simulink model "sm_pulleys_xytable_cross"  (R2026a)
settings: Solver=VariableStepAuto  StopTime=13  EnableMultiTasking=on
model workspace (MATLAB code in the model file):
  | % Pulley parameters
  | p_th  = 0.01;
  | p_gd  = 0.005;
  | p_ga  = 25;
  | p_hr  = 0.005;
  | p_rho = 7000;
  | 
  | rad_drive = 0.015*2;
  | rad_axis = 0.015*2;
  | rad_ctr = 0.015;
  | 
  | % Platform parameters
  | t_base_l = 0.4;
  | t_base_w = 0.1;
  | t_base_h = 0.01;
  | 
  | t_slider_l = 0.15;
  | t_slider_w = 0.1;
  | t_slider_h = 0.01;
  | 
  | t_pos_l = 0.025;
  | t_pos_w = 0.45;
  | t_pos_h = 0.01;
  | 
  | t_base_clr = [0.5412 0.6824 0.8392];
  | t_slider_clr = [0.635 0.984 0.498];
  | t_pos_clr = [1.0 0.99607843 0.8];
  | 
  | p_drive_clr = t_base_clr*0.8;
  | p_axis_clr = t_pos_clr*0.8;
  | p_ctr_clr = t_slider_clr*0.8;
  | 
  | 
  | 
  | p_pos_off = 0.01;
undefined symbols (not defined in the file or in its folder): Local, X, Y, Z
libraries: sm_lib x48, Multibody_Parts_Lib x15, nesl_utility x13
(part 1 of 2)
CloseFcn:
  | try,close(h1_sm_pulleys_xytable_cross),end
  | clear h1_sm_pulleys_xytable_cross
  | try,close(h2_sm_pulleys_xytable_cross),end
  | clear h2_sm_pulleys_xytable_cross
  | try,close(h3_sm_pulleys_xytable_cross),end
  | clear h3_sm_pulleys_xytable_cross
  | try,close(h4_sm_pulleys_xytable_cross),end
  | clear h4_sm_pulleys_xytable_cross
  | 
  | 
  | clear simlog_sm_pulleys_xytable_cross
  | clear logsout_sm_pulleys_xytable_cross
Description:
  | Cable-Driven XY Table with Cross Base
  | 
  | Copyright 2026 The MathWorks, Inc.
settings Model: Creator=smiller  LastModifiedBy=smiller
settings DataIOCC: SignalLoggingName=logsout_sm_pulleys_xytable_cross
settings DebuggingCC: PregeneratedLibrarySubsystemCodeDiagnostic=none
settings SimscapeCC: SimscapeNominalValues="[{\"value\":\"10\",\"unit\":\"V\"},{\"value\":\"1\",\"unit\":\"A\"},{\"value\":\"10\",\"unit\":\"N*m\"},{\"value\":\"10\",\"unit\":\"bar\"},{\"value\":\"100\",\"unit\":\"kJ/kg\"},{\"value\":\"1\",\"unit\":\"kW\"},{\"value\":\"300\",\"unit\":\"K\"},{\"value\":\"100\",\"unit\":\"cm^3/s\"},{\"value\":\"1\",\"unit\":\"kN\"},{\"value\":\"1\",\"unit\":\"g/cm^3\"},{\"value\":\"1\",\"unit\":\"l\"},{\"value\":\"1\",\"unit\":\"cm^2\"},{\"value\":\"60\",\"unit\":\"Hz\"}]"  SimscapeLogSimulationStatistics=on  SimscapeLogName=simlog_sm_pulleys_xytable_cross
settings ConfigurationSet: Description=SimMechanics 2G
settings ExplorerConfigSet: InternalSimMechanicsExplorerSettings="<ExplorerConfiguration><canonicalview>aerospace</canonicalview><AnimationSetting><BasePlaybackSpeed>1.0</BasePlaybackSpeed><PlaybackSpeedFactor>1.0</PlaybackSpeedFactor></AnimationSetting><TilePanel><TileInfo><Tiles Columns=\"1\" Count=\"2\" Rows=\"2\"><Column Weight=\"1\"/><Row Weight=\"0.6424\"/><Row Weight=\"0.3576\"/><Tile Height=\"1\" Width=\"1\" X=\"0\" Y=\"0\"/><Tile Height=\"1\" Width=\"1\" X=\"0\" Y=\"1\"/></Tiles></TileInfo><SceneInfo><SceneViewer><BGColor><R>1</R><G>1</G><B>1</B></BGColor><Camera><DoPerspective>off</DoPerspective><Position><X>1.85532256000346015e-05</X><Y>-0.00427343685538296436</Y><Z>1.02990794223546889</Z></Position><Center><X>7.04853169139587633e-06</X><Y>0.00254160839863069388</Y><Z>0.0299311649922031596</Z></Center><Up><X>0.00283398063646299022</X><Y>0.999972761893709983</Y><Z>0.00681498528375228379</Z></Up><ViewLimDist>1</ViewLimDist><YLim>0.234492363482713712</YLim><XLim>0.277049961210973916</XLim></Camera></SceneViewer><SceneViewer><BGColor><R>1</R><G>1</G><B>1</B></BGColor><Camera><DoPerspective>off</DoPerspective><Position><X>-0.689691226810977609</X><Y>-0.584891014214740101</Y><Z>0.428792646519957021</Z></Position><Center><X>0.00287853310714154473</X><Y>0.0117733409261104611</Y><Z>0.0234054551197957761</Z></Center><Up><X>0.265483592004607194</X><Y>0.311705662060663302</Y><Z>0.912336584060759237</Z></Up><ViewLimDist>1</ViewLimDist><YLim>0.103903868048192807</YLim><XLim>0.221775141309421386</XLim></Camera></SceneViewer></SceneInfo></TilePanel><MechEditorPanel><Cameras/><GfxPanelCameraMap/><VideoCreator><PlaybackSpeedRatio>1.0</PlaybackSpeedRatio><FrameRate>30</FrameRate><VideoFormat>Motion JPEG AVI</VideoFormat><FrameSize>auto</FrameSize></VideoCreator></MechEditorPanel></ExplorerConfiguration>"

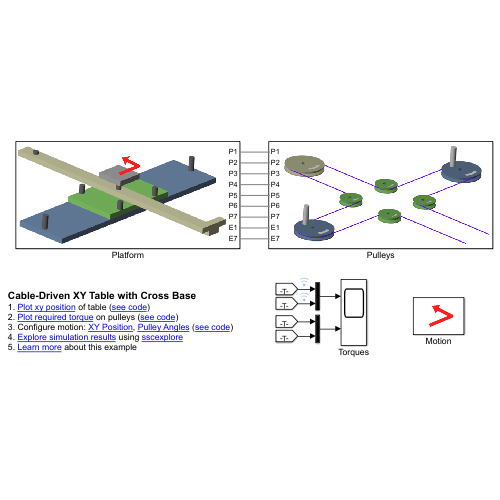
[thumbnail: Simulink's stored preview of the top-level diagram]
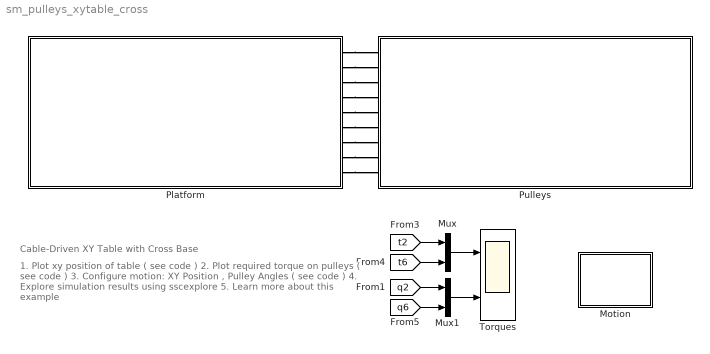
== system sm_pulleys_xytable_cross ==
  note: Cable-Driven XY Table with Cross Base
  note: 1. Plot xy position of table ( see code )
      | 2. Plot required torque on pulleys ( see code )
      | 3. Configure motion: XY Position , Pulley Angles ( see code )
      | 4. Explore simulation results using sscexplore
      | 5. Learn more about this example
  Motion : Subsystem
      mask Display: image('sm_pulleys_xytable_cross_motionXYMotion_IMAGE.png');
  Mux : Mux  Inputs=2
  Mux1 : Mux  Inputs=2
  Platform : Subsystem  Tag=PublishSubsystem
      mask Display: image('sm_pulleys_xytable_cross_platformXYMotion_IMAGE.png');
  Pulleys : Subsystem  Tag=PublishSubsystem
      mask Display: image('sm_pulleys_xytable_cross_pulleys_IMAGE.png');
  Torques : Scope  NumInputPorts=2
      settings: ActiveDisplayYMinimum=-0.14527  ActiveDisplayYMaximum=0.11195
  wires:
  [t2] -> Mux/1
  [t6] -> Mux/2
  [q2] -> Mux1/1
  [q6] -> Mux1/2
  Mux/1 -> Torques/1
  Mux1/1 -> Torques/2
  connections:
  Platform/RConn1 -- Pulleys/LConn1
  Platform/RConn2 -- Pulleys/LConn2
  Platform/RConn3 -- Pulleys/LConn3
  Platform/RConn4 -- Pulleys/LConn4
  Platform/RConn5 -- Pulleys/LConn5
  Platform/RConn6 -- Pulleys/LConn6
  Platform/RConn7 -- Pulleys/LConn7
  Platform/RConn8 -- Pulleys/LConn8
  Platform/RConn9 -- Pulleys/LConn9

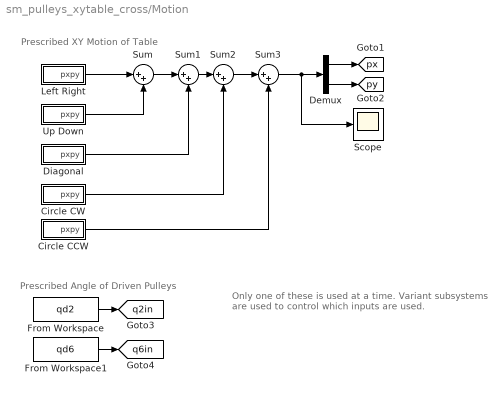
== system sm_pulleys_xytable_cross/Motion ==
  note: Only one of these is used at a time. Variant subsystems are used to control which inputs are used.
  note: Prescribed Angle of Driven Pulleys
  note: Prescribed XY Motion of Table
  Circle CCW : Subsystem
  Circle CW : Subsystem
  Demux : Demux  Outputs=2
  Diagonal : Subsystem
  From Workspace : FromWorkspace  VariableName=qd2
  From Workspace1 : FromWorkspace  VariableName=qd6
  Left Right : Subsystem
  Scope : Scope
      settings: ActiveDisplayYMinimum=-0.125  ActiveDisplayYMaximum=0.125
  Sum{,1..3} (4 alike) : Sum  Inputs=|++
  Up Down : Subsystem
  tag scope: px=global, py=global, q2in=global, q6in=global
  wires:
  Demux/1 -> [px]
  Demux/2 -> [py]
  Sum3/1 -> Scope/1, Demux/1
  Left Right/1(pxpy) -> Sum/1
  Diagonal/1(pxpy) -> Sum1/2
  Sum/1 -> Sum1/1
  Up Down/1(pxpy) -> Sum/2
  Sum1/1 -> Sum2/1
  Circle CW/1(pxpy) -> Sum2/2
  From Workspace/1 -> [q2in]
  From Workspace1/1 -> [q6in]
  Sum2/1 -> Sum3/1
  Circle CCW/1(pxpy) -> Sum3/2

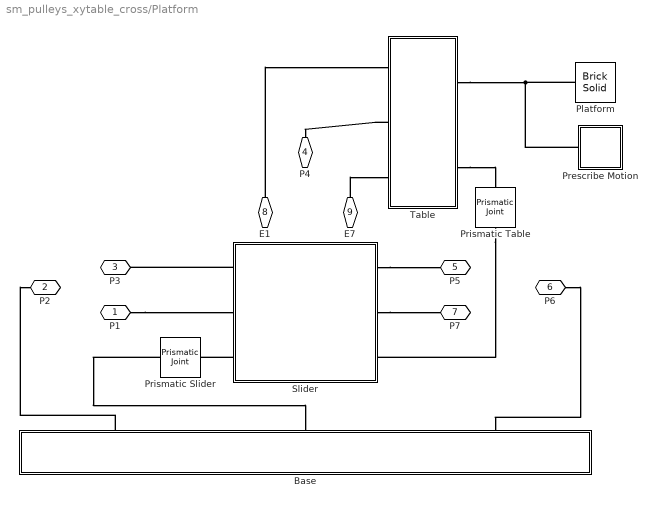
== system sm_pulleys_xytable_cross/Platform ==
  Base : Subsystem
      mask Display: image('sm_pulleys_xytable_cross_base_IMAGE.png');
  Platform : sm_lib/Body Elements/Brick Solid  BrickDimensions=[0.05 0.05 0.01]  BrickDimensionsUnits=m  ExportEntireGeometry=off  InertiaType=CalculateFromGeometry  BasedOnType=Density  Density=1000  DensityUnits=kg/m^3  Mass=1  MassUnits=kg  CenterOfMass=[0 0 0]  CenterOfMassUnits=m  MomentsOfInertia=[1 1 1]  MomentsOfInertiaUnits=kg*m^2  ProductsOfInertia=[0 0 0]  ProductsOfInertiaUnits=kg*m^2  GraphicType=FromGeometry  MarkerShape=Sphere  MarkerSize=10  GraphicVisPropType=SimpleVisualProperties  GraphicDiffuseColor=[0.8 0.8 0.8]  GraphicOpacity=1.0  GraphicSpecularColor=[0.5 0.5 0.5 1.0]  GraphicAmbientColor=[0.15 0.15 0.15 1.0]  GraphicEmissiveColor=[0.0 0.0 0.0 1.0]  GraphicShininess=75  DoExposeReferenceFrame=off  SerializedFrames=<Frames><Frame><Id>Frame1</Id><Value><Name>T</Name><Origin><Source>GeometricFeature</Source><FeatureName>+z surface</FeatureName></Origin><PrimaryAxis><DefinedDirection>+Z</DefinedDirection><Source>ReferenceFrame</Source><SourceDirection>+Z</SourceDirection><FeatureName></FeatureName></PrimaryAxis><SecondaryAxis><DefinedDirection>+X</DefinedDirection><Source>ReferenceFrame</Source><SourceDirection>+X</SourceDirection><FeatureName></FeatureName></SecondaryAxis></Value></Frame><Frame><Id>Frame2</Id><Value><Name>B</Name><Origin><Source>GeometricFeature</Source><FeatureName>-z surface</FeatureName></Origin><PrimaryAxis><DefinedDirection>+Z</DefinedDirection><Source>ReferenceFrame</Source><SourceDirection>+Z</SourceDirection><FeatureName></FeatureName></PrimaryAxis><SecondaryAxis><DefinedDirection>+X</DefinedDirection><Source>ReferenceFrame</Source><SourceDirection>+X</SourceDirection><FeatureName></FeatureName></SecondaryAxis></Value></Frame></Frames>
  Prescribe Motion : Subsystem  Variant=on  VariantControlMode=label  VariantControl=Variant1  LabelModeActiveChoice=On
      settings: AttributesFormatString=%<ActiveVariant>
      mask Display:
      | blk = Multibody_Parts_Library_activeVariantBlock(gcb);
      | eval(get_param(blk, 'MaskDisplay'));
  Prismatic Table : sm_lib/Joints/Prismatic Joint  JointMode=Normal  CompositeWrenchDir=FollowerOnBase  CompositeWrenchFrame=BaseFrame  SenseConstraintForce=off  SenseConstraintTorque=off  SenseTotalForce=off  SenseTotalTorque=off  PositionTargetSpecify=off  PositionTargetPriority=High  PositionTargetValue=0  PositionTargetValueUnits=m  VelocityTargetSpecify=off  VelocityTargetPriority=High  VelocityTargetValue=0  VelocityTargetValueUnits=m/s  EquilibriumPosition=0  EquilibriumPositionUnits=m  SpringStiffness=0  SpringStiffnessUnits=N/m  DampingCoefficient=0  DampingCoefficientUnits=N/(m/s)  LowerLimitSpecify=off  LowerLimitBound=-1  LowerLimitBoundUnits=m  LowerLimitStiffness=1e6  LowerLimitStiffnessUnits=N/m  LowerLimitDamping=1e3  LowerLimitDampingUnits=N/(m/s)  LowerLimitTransitionRegionWidth=1e-4  LowerLimitTransitionRegionWidthUnits=m  UpperLimitSpecify=off  UpperLimitBound=1  UpperLimitBoundUnits=m  UpperLimitStiffness=1e6  UpperLimitStiffnessUnits=N/m  UpperLimitDamping=1e3  UpperLimitDampingUnits=N/(m/s)  UpperLimitTransitionRegionWidth=1e-4  UpperLimitTransitionRegionWidthUnits=m  TorqueActuationMode=NoTorque  MotionActuationMode=ComputedMotion  SensePosition=off  SenseVelocity=off  SenseAcceleration=off  SenseTorqueForce=off  SenseLowerLimitTorqueForce=off  SenseUpperLimitTorqueForce=off
  Prismatic Slider : sm_lib/Joints/Prismatic Joint  JointMode=Normal  CompositeWrenchDir=FollowerOnBase  CompositeWrenchFrame=BaseFrame  SenseConstraintForce=off  SenseConstraintTorque=off  SenseTotalForce=off  SenseTotalTorque=off  PositionTargetSpecify=off  PositionTargetPriority=High  PositionTargetValue=0  PositionTargetValueUnits=m  VelocityTargetSpecify=off  VelocityTargetPriority=High  VelocityTargetValue=0  VelocityTargetValueUnits=m/s  EquilibriumPosition=0  EquilibriumPositionUnits=m  SpringStiffness=0  SpringStiffnessUnits=N/m  DampingCoefficient=0  DampingCoefficientUnits=N/(m/s)  LowerLimitSpecify=off  LowerLimitBound=-1  LowerLimitBoundUnits=m  LowerLimitStiffness=1e6  LowerLimitStiffnessUnits=N/m  LowerLimitDamping=1e3  LowerLimitDampingUnits=N/(m/s)  LowerLimitTransitionRegionWidth=1e-4  LowerLimitTransitionRegionWidthUnits=m  UpperLimitSpecify=off  UpperLimitBound=1  UpperLimitBoundUnits=m  UpperLimitStiffness=1e6  UpperLimitStiffnessUnits=N/m  UpperLimitDamping=1e3  UpperLimitDampingUnits=N/(m/s)  UpperLimitTransitionRegionWidth=1e-4  UpperLimitTransitionRegionWidthUnits=m  TorqueActuationMode=NoTorque  MotionActuationMode=ComputedMotion  SensePosition=off  SenseVelocity=off  SenseAcceleration=off  SenseTorqueForce=off  SenseLowerLimitTorqueForce=off  SenseUpperLimitTorqueForce=off
  Slider : Subsystem
      mask Display: image('sm_pulleys_xytable_cross_slider_IMAGE.png');
  Table : Subsystem
      mask Display: image('sm_pulleys_xytable_cross_table_IMAGE.png')
  P1 : PMIOPort  Side=Right
  P2 : PMIOPort  Port=2  Side=Right
  P3 : PMIOPort  Port=3  Side=Right
  P4 : PMIOPort  Port=4  Side=Right
  P5 : PMIOPort  Port=5  Side=Right
  P6 : PMIOPort  Port=6  Side=Right
  P7 : PMIOPort  Port=7  Side=Right
  E1 : PMIOPort  Port=8  Side=Right
  E7 : PMIOPort  Port=9  Side=Right
  connections:
  E1/RConn1 -- Table/LConn1
  E7/RConn1 -- Table/LConn3
  Table/LConn2 -- P4/RConn1
  Table/RConn2 -- Prismatic Table/RConn1
  Prismatic Table/LConn1 -- Slider/RConn3
  Slider/LConn3 -- Prismatic Slider/RConn1
  P1/RConn1 -- Slider/LConn2
  Prismatic Slider/LConn1 -- Base/RConn2
  P6/RConn1 -- Base/RConn3
  Slider/RConn1 -- P5/RConn1
  Slider/LConn1 -- P3/RConn1
  Slider/RConn2 -- P7/RConn1
  Base/RConn1 -- P2/RConn1
  Platform/RConn1 -- Table/RConn1 -- Prescribe Motion/RConn1

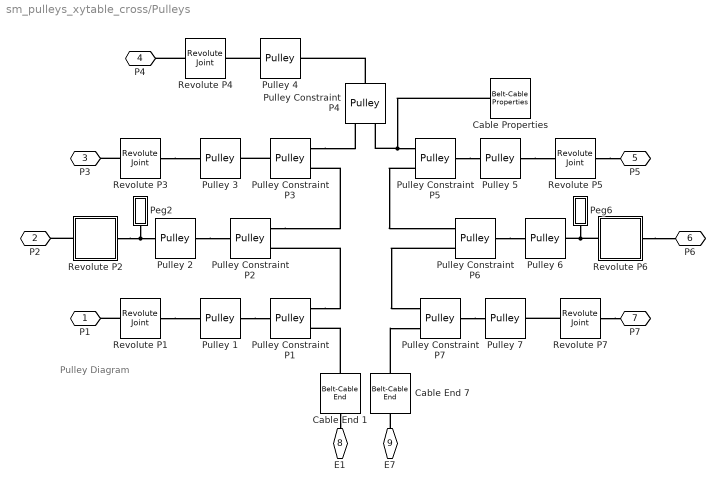
== system sm_pulleys_xytable_cross/Pulleys ==
  note: Pulley
      | Diagram
  Cable End 1 : sm_lib/Belts and Cables/Belt-Cable End
  Cable End 7 : sm_lib/Belts and Cables/Belt-Cable End
  Cable Properties : sm_lib/Belts and Cables/Belt-Cable Properties  DrumBeltCableAlignment=MonitoredPlanar  GraphicType=PitchLine  GraphicVisPropType=SimpleVisualProperties  GraphicDiffuseColor=[0.4 0.0 1.0]  GraphicOpacity=1.0  GraphicSpecularColor=[0.5 0.5 0.5 1.0]  GraphicAmbientColor=[0.15 0.15 0.15 1.0]  GraphicEmissiveColor=[0.0 0.0 0.0 1.0]  GraphicShininess=75
  Peg2 : Subsystem
  Peg6 : Subsystem
  Pulley Constraint P{1,3,5,7} (4 alike) : sm_lib/Belts and Cables/Pulley  PitchRadius=rad_ctr  PitchRadiusUnits=m  InitialWrapAngleLowerBound=0.0  InitialWrapAngleLowerBoundUnits=deg  SenseWrapAngle=off  SensePulleyAngleA=off  SensePulleyAngleB=off  SenseFleetAngleA=off  SenseFleetAngleB=off
  Pulley Constraint P2 : sm_lib/Belts and Cables/Pulley  PitchRadius=rad_drive  PitchRadiusUnits=m  InitialWrapAngleLowerBound=0.0  InitialWrapAngleLowerBoundUnits=deg  SenseWrapAngle=off  SensePulleyAngleA=off  SensePulleyAngleB=off  SenseFleetAngleA=off  SenseFleetAngleB=off
  Pulley Constraint P4 : sm_lib/Belts and Cables/Pulley  PitchRadius=rad_axis  PitchRadiusUnits=m  InitialWrapAngleLowerBound=0.0  InitialWrapAngleLowerBoundUnits=deg  SenseWrapAngle=off  SensePulleyAngleA=off  SensePulleyAngleB=off  SenseFleetAngleA=off  SenseFleetAngleB=off
  Pulley Constraint P6 : sm_lib/Belts and Cables/Pulley  PitchRadius=rad_drive  PitchRadiusUnits=m  InitialWrapAngleLowerBound=0.0  InitialWrapAngleLowerBoundUnits=deg  SenseWrapAngle=off  SensePulleyAngleA=off  SensePulleyAngleB=off  SenseFleetAngleA=off  SenseFleetAngleB=off
  Pulley 1 : Multibody_Parts_Lib/Basic/Pulley  pulley_rad=rad_ctr  pulley_d_grv=p_gd  pulley_a_grv=p_ga  pulley_th=p_th  pulley_radh=p_hr  pulley_rho=p_rho  pulley_clr=p_ctr_clr  pulley_opc=1  pulley_zori=Yes, about X  popup_markings=One  mark_radius_range=[0.7 0.9]  mark_angle_range=60  mark_color=[1 1 1]
      settings: SourceProductName=Simscape Multibody Parts Library
  Pulley 2 : Multibody_Parts_Lib/Basic/Pulley  pulley_rad=rad_drive  pulley_d_grv=p_gd  pulley_a_grv=p_ga  pulley_th=p_th  pulley_radh=p_hr  pulley_rho=p_rho  pulley_clr=p_drive_clr  pulley_opc=1  pulley_zori=No  popup_markings=One  mark_radius_range=[0.7 0.9]  mark_angle_range=60  mark_color=[1 1 1]
      settings: SourceProductName=Simscape Multibody Parts Library
  Pulley 3 : Multibody_Parts_Lib/Basic/Pulley  pulley_rad=rad_ctr  pulley_d_grv=p_gd  pulley_a_grv=p_ga  pulley_th=p_th  pulley_radh=p_hr  pulley_rho=p_rho  pulley_clr=p_ctr_clr  pulley_opc=1  pulley_zori=Yes, about X  popup_markings=One  mark_radius_range=[0.7 0.9]  mark_angle_range=60  mark_color=[1 1 1]
      settings: SourceProductName=Simscape Multibody Parts Library
  Pulley 4 : Multibody_Parts_Lib/Basic/Pulley  pulley_rad=rad_axis  pulley_d_grv=p_gd  pulley_a_grv=p_ga  pulley_th=p_th  pulley_radh=p_hr  pulley_rho=p_rho  pulley_clr=p_axis_clr  pulley_opc=1  pulley_zori=Yes, about X  popup_markings=One  mark_radius_range=[0.7 0.9]  mark_angle_range=60  mark_color=[1 1 1]
      settings: SourceProductName=Simscape Multibody Parts Library
  Pulley 5 : Multibody_Parts_Lib/Basic/Pulley  pulley_rad=rad_ctr  pulley_d_grv=p_gd  pulley_a_grv=p_ga  pulley_th=p_th  pulley_radh=p_hr  pulley_rho=p_rho  pulley_clr=p_ctr_clr  pulley_opc=1  pulley_zori=No  popup_markings=One  mark_radius_range=[0.7 0.9]  mark_angle_range=60  mark_color=[1 1 1]
      settings: SourceProductName=Simscape Multibody Parts Library
  Pulley 6 : Multibody_Parts_Lib/Basic/Pulley  pulley_rad=rad_drive  pulley_d_grv=p_gd  pulley_a_grv=p_ga  pulley_th=p_th  pulley_radh=p_hr  pulley_rho=p_rho  pulley_clr=p_drive_clr  pulley_opc=1  pulley_zori=Yes, about X  popup_markings=One  mark_radius_range=[0.7 0.9]  mark_angle_range=60  mark_color=[1 1 1]
      settings: SourceProductName=Simscape Multibody Parts Library
  Pulley 7 : Multibody_Parts_Lib/Basic/Pulley  pulley_rad=rad_ctr  pulley_d_grv=p_gd  pulley_a_grv=p_ga  pulley_th=p_th  pulley_radh=p_hr  pulley_rho=p_rho  pulley_clr=p_ctr_clr  pulley_opc=1  pulley_zori=No  popup_markings=One  mark_radius_range=[0.7 0.9]  mark_angle_range=60  mark_color=[1 1 1]
      settings: SourceProductName=Simscape Multibody Parts Library
  Revolute P{1,3..5,7} (5 alike) : sm_lib/Joints/Revolute Joint  JointMode=Normal  CompositeWrenchDir=FollowerOnBase  CompositeWrenchFrame=BaseFrame  SenseConstraintForce=off  SenseConstraintTorque=off  SenseTotalForce=off  SenseTotalTorque=off  PositionTargetSpecify=off  PositionTargetPriority=High  PositionTargetValue=0  PositionTargetValueUnits=deg  VelocityTargetSpecify=off  VelocityTargetPriority=High  VelocityTargetValue=0  VelocityTargetValueUnits=deg/s  EquilibriumPosition=0  EquilibriumPositionUnits=deg  SpringStiffness=0  SpringStiffnessUnits=N*m/deg  DampingCoefficient=0  DampingCoefficientUnits=N*m/(deg/s)  LowerLimitSpecify=off  LowerLimitBound=-90  LowerLimitBoundUnits=deg  LowerLimitStiffness=1e4  LowerLimitStiffnessUnits=N*m/deg  LowerLimitDamping=10  LowerLimitDampingUnits=N*m/(deg/s)  LowerLimitTransitionRegionWidth=0.1  LowerLimitTransitionRegionWidthUnits=deg  UpperLimitSpecify=off  UpperLimitBound=90  UpperLimitBoundUnits=deg  UpperLimitStiffness=1e4  UpperLimitStiffnessUnits=N*m/deg  UpperLimitDamping=10  UpperLimitDampingUnits=N*m/(deg/s)  UpperLimitTransitionRegionWidth=0.1  UpperLimitTransitionRegionWidthUnits=deg  TorqueActuationMode=NoTorque  MotionActuationMode=ComputedMotion  SensePosition=off  SenseVelocity=off  SenseAcceleration=off  SenseTorqueForce=off  SenseLowerLimitTorqueForce=off  SenseUpperLimitTorqueForce=off
  Revolute P2 : Subsystem  Variant=on  VariantControlMode=label  VariantControl=Variant1  LabelModeActiveChoice=Measure
      settings: AttributesFormatString=%<ActiveVariant>
      mask Display:
      | blk = Multibody_Parts_Library_activeVariantBlock(gcb);
      | eval(get_param(blk, 'MaskDisplay'));
  Revolute P6 : Subsystem  Variant=on  VariantControlMode=label  VariantControl=Variant1  LabelModeActiveChoice=Measure
      settings: AttributesFormatString=%<ActiveVariant>
      mask Display:
      | blk = Multibody_Parts_Library_activeVariantBlock(gcb);
      | eval(get_param(blk, 'MaskDisplay'));
  P1 : PMIOPort  Side=Left
  P2 : PMIOPort  Port=2  Side=Left
  P3 : PMIOPort  Port=3  Side=Left
  P4 : PMIOPort  Port=4  Side=Left
  P5 : PMIOPort  Port=5  Side=Left
  P6 : PMIOPort  Port=6  Side=Left
  P7 : PMIOPort  Port=7  Side=Left
  E1 : PMIOPort  Port=8  Side=Left
  E7 : PMIOPort  Port=9  Side=Left
  connections:
  Revolute P1/LConn1 -- P1/RConn1
  Revolute P1/RConn1 -- Pulley 1/LConn1
  Cable End 1/LConn1 -- E1/RConn1
  Revolute P3/RConn1 -- Pulley 3/LConn1
  Pulley Constraint P3/LConn1 -- Pulley 3/RConn1
  Revolute P4/LConn1 -- P4/RConn1
  Pulley 4/LConn1 -- Revolute P4/RConn1
  Pulley Constraint P4/LConn1 -- Pulley 4/RConn1
  Revolute P5/LConn1 -- P5/RConn1
  Pulley 5/LConn1 -- Revolute P5/RConn1
  Pulley Constraint P5/LConn1 -- Pulley 5/RConn1
  Pulley Constraint P6/LConn1 -- Pulley 6/RConn1
  Pulley Constraint P5/RConn2 -- Pulley Constraint P6/RConn1
  Revolute P7/LConn1 -- P7/RConn1
  Revolute P7/RConn1 -- Pulley 7/RConn1
  Pulley Constraint P7/LConn1 -- Pulley 7/LConn1
  E7/RConn1 -- Cable End 7/LConn1
  Cable End 7/RConn1 -- Pulley Constraint P7/RConn2
  Revolute P3/LConn1 -- P3/RConn1
  Cable End 1/RConn1 -- Pulley Constraint P1/RConn2
  Pulley Constraint P1/RConn1 -- Pulley Constraint P2/RConn2
  Pulley Constraint P2/RConn1 -- Pulley Constraint P3/RConn2
  Pulley Constraint P3/RConn1 -- Pulley Constraint P4/RConn1
  Cable Properties/LConn1 -- Pulley Constraint P4/RConn2 -- Pulley Constraint P5/RConn1
  Pulley Constraint P6/RConn2 -- Pulley Constraint P7/RConn1
  Pulley 2/RConn1 -- Pulley Constraint P2/LConn1
  Pulley 1/RConn1 -- Pulley Constraint P1/LConn1
  Revolute P2/LConn1 -- P2/RConn1
  Revolute P2/RConn1 -- Peg2/RConn1 -- Pulley 2/LConn1
  Revolute P6/LConn1 -- P6/RConn1
  Revolute P6/RConn1 -- Peg6/RConn1 -- Pulley 6/LConn1

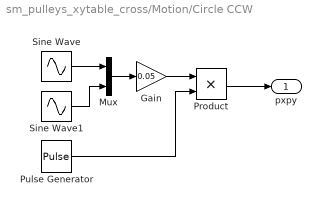
== system sm_pulleys_xytable_cross/Motion/Circle CCW ==
  Gain : Gain  Gain=0.05
  Mux : Mux  Inputs=2
  Product : Product
  Pulse Generator : DiscretePulseGenerator  PulseType=Time based  Period=15  PulseWidth=16.667  PhaseDelay=10
  Sine Wave : Sin  Bias=-1  Frequency=2*pi/2.5  Phase=pi/2  SampleTime=0
  Sine Wave1 : Sin  Frequency=2*pi/2.5  SampleTime=0
  pxpy : Outport  VectorParamsAs1DForOutWhenUnconnected=off
  wires:
  Product/1 -> pxpy/1
  Sine Wave1/1 -> Mux/2
  Pulse Generator/1 -> Product/2
  Mux/1 -> Gain/1
  Gain/1 -> Product/1
  Sine Wave/1 -> Mux/1

== system sm_pulleys_xytable_cross/Motion/Circle CW ==
  Gain : Gain  Gain=0.05
  Mux : Mux  Inputs=2
  Product : Product
  Pulse Generator : DiscretePulseGenerator  PulseType=Time based  Period=15  PulseWidth=16.667  PhaseDelay=7.5
  Sine Wave : Sin  Bias=1  Frequency=2*pi/2.5  Phase=3*pi/2  SampleTime=0
  Sine Wave1 : Sin  Frequency=2*pi/2.5  SampleTime=0
  pxpy : Outport  VectorParamsAs1DForOutWhenUnconnected=off
  wires:
  Sine Wave/1 -> Mux/1
  Gain/1 -> Product/1
  Mux/1 -> Gain/1
  Pulse Generator/1 -> Product/2
  Sine Wave1/1 -> Mux/2
  Product/1 -> pxpy/1

== system sm_pulleys_xytable_cross/Motion/Diagonal ==
  Gain : Gain  Gain=0.05
  Mux : Mux  Inputs=2
  Product : Product
  Pulse Generator : DiscretePulseGenerator  PulseType=Time based  Period=15  PulseWidth=16.667  PhaseDelay=5
  Sine Wave : Sin  Frequency=2*pi/2.5  SampleTime=0
  Sine Wave1 : Sin  Frequency=2*pi/2.5  SampleTime=0
  pxpy : Outport  VectorParamsAs1DForOutWhenUnconnected=off
  wires:
  Product/1 -> pxpy/1
  Sine Wave1/1 -> Mux/2
  Pulse Generator/1 -> Product/2
  Mux/1 -> Gain/1
  Gain/1 -> Product/1
  Sine Wave/1 -> Mux/1

== system sm_pulleys_xytable_cross/Motion/Left Right ==
  Gain : Gain  Gain=0.05
  Mux : Mux  Inputs=2
  Product : Product
  Pulse Generator : DiscretePulseGenerator  PulseType=Time based  Period=15  PulseWidth=16.667
  Sine Wave : Sin  Frequency=2*pi/2.5  SampleTime=0
  Sine Wave1 : Sin  Amplitude=-1*0  Frequency=2*pi/2.5  SampleTime=0
  pxpy : Outport  VectorParamsAs1DForOutWhenUnconnected=off
  wires:
  Sine Wave/1 -> Mux/1
  Gain/1 -> Product/1
  Mux/1 -> Gain/1
  Pulse Generator/1 -> Product/2
  Sine Wave1/1 -> Mux/2
  Product/1 -> pxpy/1

== system sm_pulleys_xytable_cross/Motion/Up Down ==
  Gain : Gain  Gain=0.05
  Mux : Mux  Inputs=2
  Product : Product
  Pulse Generator : DiscretePulseGenerator  PulseType=Time based  Period=15  PulseWidth=16.667  PhaseDelay=2.5
  Sine Wave : Sin  Amplitude=1*0  Frequency=2*pi/2.5  SampleTime=0
  Sine Wave1 : Sin  Frequency=2*pi/2.5  SampleTime=0
  pxpy : Outport  VectorParamsAs1DForOutWhenUnconnected=off
  wires:
  Product/1 -> pxpy/1
  Sine Wave1/1 -> Mux/2
  Pulse Generator/1 -> Product/2
  Mux/1 -> Gain/1
  Gain/1 -> Product/1
  Sine Wave/1 -> Mux/1

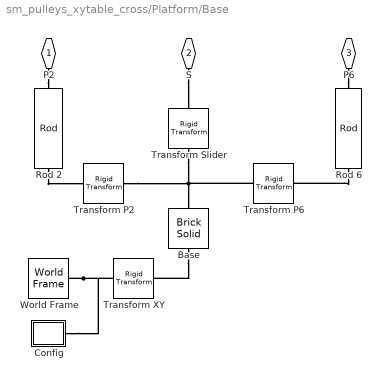
== system sm_pulleys_xytable_cross/Platform/Base ==
  Base : sm_lib/Body Elements/Brick Solid  BrickDimensions=[t_base_w t_base_l t_base_h]  BrickDimensionsUnits=m  ExportEntireGeometry=off  InertiaType=CalculateFromGeometry  BasedOnType=Density  Density=1000  DensityUnits=kg/m^3  Mass=1  MassUnits=kg  CenterOfMass=[0 0 0]  CenterOfMassUnits=m  MomentsOfInertia=[1 1 1]  MomentsOfInertiaUnits=kg*m^2  ProductsOfInertia=[0 0 0]  ProductsOfInertiaUnits=kg*m^2  GraphicType=FromGeometry  MarkerShape=Sphere  MarkerSize=10  GraphicVisPropType=SimpleVisualProperties  GraphicDiffuseColor=t_base_clr  GraphicOpacity=1.0  GraphicSpecularColor=[0.5 0.5 0.5 1.0]  GraphicAmbientColor=[0.15 0.15 0.15 1.0]  GraphicEmissiveColor=[0.0 0.0 0.0 1.0]  GraphicShininess=128  DoExposeReferenceFrame=off  SerializedFrames=<Frames><Frame><Id>Frame1</Id><Value><Name>T</Name><Origin><Source>GeometricFeature</Source><FeatureName>+z surface</FeatureName></Origin><PrimaryAxis><DefinedDirection>+Z</DefinedDirection><Source>ReferenceFrame</Source><SourceDirection>+Z</SourceDirection><FeatureName></FeatureName></PrimaryAxis><SecondaryAxis><DefinedDirection>+X</DefinedDirection><Source>ReferenceFrame</Source><SourceDirection>+X</SourceDirection><FeatureName></FeatureName></SecondaryAxis></Value></Frame><Frame><Id>Frame2</Id><Value><Name>B</Name><Origin><Source>GeometricFeature</Source><FeatureName>-z surface</FeatureName></Origin><PrimaryAxis><DefinedDirection>+Z</DefinedDirection><Source>ReferenceFrame</Source><SourceDirection>+Z</SourceDirection><FeatureName></FeatureName></PrimaryAxis><SecondaryAxis><DefinedDirection>+X</DefinedDirection><Source>ReferenceFrame</Source><SourceDirection>+X</SourceDirection><FeatureName></FeatureName></SecondaryAxis></Value></Frame></Frames>
  Config : Subsystem
  Rod 2 : Multibody_Parts_Lib/Basic/Rod  rod_rad=p_hr  rod_len=t_slider_h+t_pos_h+p_th/2  rod_rho=7000  rod_color=[0.5 0.5 0.5]  rod_opc=1  popup_zori=Local +Z  popup_markings=None  mark_radius_range=[0.5 1.01]  mark_length_range=1.005  mark_angle_range=30  mark_color=[1 1 1]
      settings: SourceProductName=Simscape Multibody Parts Library
  Rod 6 : Multibody_Parts_Lib/Basic/Rod  rod_rad=p_hr  rod_len=t_slider_h+t_pos_h+p_th/2  rod_rho=7000  rod_color=[0.5 0.5 0.5]  rod_opc=1  popup_zori=Local +Z  popup_markings=None  mark_radius_range=[0.5 1.01]  mark_length_range=1.005  mark_angle_range=30  mark_color=[1 1 1]
      settings: SourceProductName=Simscape Multibody Parts Library
  Transform Slider : sm_lib/Frames and Transforms/Rigid Transform  RotationMethod=StandardAxis  FollAlignAxisA=+X  BaseAlignAxisA=+Y  FollAlignAxisB=+Y  BaseAlignAxisB=+Z  RotationStandardAxis=-X  RotationAngle=90  RotationAngleUnits=deg  RotationArbitraryAxis=[0 0 1]  RotationSequenceAxes=FollowerAxes  RotationSequence=XYX  RotationSequenceAngles=[0 0 0]  RotationSequenceAnglesUnits=deg  RotationMatrix=[1 0 0; 0 1 0; 0 0 1]  Quaternion=[1 0 0 0]  TranslationMethod=None  TranslationCartesianOffset=[0 0 0]  TranslationCartesianOffsetUnits=m  TranslationStandardAxis=+Z  TranslationStandardOffset=0  TranslationStandardOffsetUnits=m  TranslationROffset=0  TranslationROffsetUnits=m  TranslationThetaOffset=0  TranslationThetaOffsetUnits=deg  TranslationZOffset=0  TranslationZOffsetUnits=m
  Transform XY : sm_lib/Frames and Transforms/Rigid Transform  RotationMethod=StandardAxis  FollAlignAxisA=+X  BaseAlignAxisA=+Y  FollAlignAxisB=+Y  BaseAlignAxisB=+Z  RotationStandardAxis=+Z  RotationAngle=-90  RotationAngleUnits=deg  RotationArbitraryAxis=[0 0 1]  RotationSequenceAxes=FollowerAxes  RotationSequence=XYX  RotationSequenceAngles=[0 0 0]  RotationSequenceAnglesUnits=deg  RotationMatrix=[1 0 0; 0 1 0; 0 0 1]  Quaternion=[1 0 0 0]  TranslationMethod=None  TranslationCartesianOffset=[0 0 0]  TranslationCartesianOffsetUnits=m  TranslationStandardAxis=+Z  TranslationStandardOffset=0  TranslationStandardOffsetUnits=m  TranslationROffset=0  TranslationROffsetUnits=m  TranslationThetaOffset=0  TranslationThetaOffsetUnits=deg  TranslationZOffset=0  TranslationZOffsetUnits=m
  Transform P6 : sm_lib/Frames and Transforms/Rigid Transform  RotationMethod=None  FollAlignAxisA=+X  BaseAlignAxisA=+Y  FollAlignAxisB=+Y  BaseAlignAxisB=+Z  RotationStandardAxis=+Z  RotationAngle=0.0  RotationAngleUnits=deg  RotationArbitraryAxis=[0 0 1]  RotationSequenceAxes=FollowerAxes  RotationSequence=XYX  RotationSequenceAngles=[0 0 0]  RotationSequenceAnglesUnits=deg  RotationMatrix=[1 0 0; 0 1 0; 0 0 1]  Quaternion=[1 0 0 0]  TranslationMethod=StandardAxis  TranslationCartesianOffset=[0 0 0]  TranslationCartesianOffsetUnits=m  TranslationStandardAxis=+Y  TranslationStandardOffset=t_base_l/2-p_hr*2  TranslationStandardOffsetUnits=m  TranslationROffset=0  TranslationROffsetUnits=m  TranslationThetaOffset=0  TranslationThetaOffsetUnits=deg  TranslationZOffset=0  TranslationZOffsetUnits=m
  Transform P2 : sm_lib/Frames and Transforms/Rigid Transform  RotationMethod=None  FollAlignAxisA=+X  BaseAlignAxisA=+Y  FollAlignAxisB=+Y  BaseAlignAxisB=+Z  RotationStandardAxis=+Z  RotationAngle=0.0  RotationAngleUnits=deg  RotationArbitraryAxis=[0 0 1]  RotationSequenceAxes=FollowerAxes  RotationSequence=XYX  RotationSequenceAngles=[0 0 0]  RotationSequenceAnglesUnits=deg  RotationMatrix=[1 0 0; 0 1 0; 0 0 1]  Quaternion=[1 0 0 0]  TranslationMethod=StandardAxis  TranslationCartesianOffset=[0 0 0]  TranslationCartesianOffsetUnits=m  TranslationStandardAxis=-Y  TranslationStandardOffset=t_base_l/2-p_hr*2  TranslationStandardOffsetUnits=m  TranslationROffset=0  TranslationROffsetUnits=m  TranslationThetaOffset=0  TranslationThetaOffsetUnits=deg  TranslationZOffset=0  TranslationZOffsetUnits=m
  World Frame : sm_lib/Frames and Transforms/World Frame
  P2 : PMIOPort  Side=Right
  S : PMIOPort  Port=2  Side=Right
  P6 : PMIOPort  Port=3  Side=Right
  connections:
  World Frame/RConn1 -- Transform XY/LConn1 -- Config/RConn1
  P6/RConn1 -- Rod 6/RConn1
  P2/RConn1 -- Rod 2/RConn1
  Transform Slider/LConn1 -- Transform P6/LConn1 -- Transform P2/LConn1 -- Base/LConn1
  S/RConn1 -- Transform Slider/RConn1
  Base/RConn1 -- Transform XY/RConn1
  Rod 6/LConn1 -- Transform P6/RConn1
  Rod 2/LConn1 -- Transform P2/RConn1

== system sm_pulleys_xytable_cross/Platform/Prescribe Motion ==
  Off : Subsystem  Tag=PublishSubsystem  VariantControl=Off
      mask Display: image('sm_pulleys_xytable_cross_prescribeMotionOff_IMAGE.png')
  On : Subsystem  Tag=PublishSubsystem  VariantControl=On
      mask Display: image('sm_pulleys_xytable_cross_prescribeMotionOn_IMAGE.png')
  " F" : PMIOPort  Side=Right

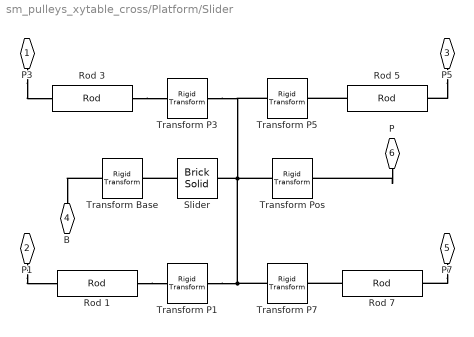
== system sm_pulleys_xytable_cross/Platform/Slider ==
  Rod {1,3,5,7} (4 alike) : Multibody_Parts_Lib/Basic/Rod  rod_rad=p_hr  rod_len=t_pos_h+p_th/2  rod_rho=7000  rod_color=[0.5 0.5 0.5]  rod_opc=1  popup_zori=Local +Z  popup_markings=None  mark_radius_range=[0.5 1.01]  mark_length_range=1.005  mark_angle_range=30  mark_color=[1 1 1]
      settings: SourceProductName=Simscape Multibody Parts Library
  Slider : sm_lib/Body Elements/Brick Solid  BrickDimensions=[t_slider_w t_slider_l t_slider_h]  BrickDimensionsUnits=m  ExportEntireGeometry=off  InertiaType=CalculateFromGeometry  BasedOnType=Density  Density=1000  DensityUnits=kg/m^3  Mass=1  MassUnits=kg  CenterOfMass=[0 0 0]  CenterOfMassUnits=m  MomentsOfInertia=[1 1 1]  MomentsOfInertiaUnits=kg*m^2  ProductsOfInertia=[0 0 0]  ProductsOfInertiaUnits=kg*m^2  GraphicType=FromGeometry  MarkerShape=Sphere  MarkerSize=10  GraphicVisPropType=SimpleVisualProperties  GraphicDiffuseColor=t_slider_clr  GraphicOpacity=1.0  GraphicSpecularColor=[0.5 0.5 0.5 1.0]  GraphicAmbientColor=[0.15 0.15 0.15 1.0]  GraphicEmissiveColor=[0.0 0.0 0.0 1.0]  GraphicShininess=75  DoExposeReferenceFrame=off  SerializedFrames=<Frames><Frame><Id>Frame1</Id><Value><Name>T</Name><Origin><Source>GeometricFeature</Source><FeatureName>+z surface</FeatureName></Origin><PrimaryAxis><DefinedDirection>+Z</DefinedDirection><Source>ReferenceFrame</Source><SourceDirection>+Z</SourceDirection><FeatureName></FeatureName></PrimaryAxis><SecondaryAxis><DefinedDirection>+X</DefinedDirection><Source>ReferenceFrame</Source><SourceDirection>+X</SourceDirection><FeatureName></FeatureName></SecondaryAxis></Value></Frame><Frame><Id>Frame2</Id><Value><Name>B</Name><Origin><Source>GeometricFeature</Source><FeatureName>-z surface</FeatureName></Origin><PrimaryAxis><DefinedDirection>+Z</DefinedDirection><Source>ReferenceFrame</Source><SourceDirection>+Z</SourceDirection><FeatureName></FeatureName></PrimaryAxis><SecondaryAxis><DefinedDirection>+X</DefinedDirection><Source>ReferenceFrame</Source><SourceDirection>+X</SourceDirection><FeatureName></FeatureName></SecondaryAxis></Value></Frame></Frames>
  Transform Base : sm_lib/Frames and Transforms/Rigid Transform  RotationMethod=StandardAxis  FollAlignAxisA=+X  BaseAlignAxisA=+Y  FollAlignAxisB=+Y  BaseAlignAxisB=+Z  RotationStandardAxis=+X  RotationAngle=90  RotationAngleUnits=deg  RotationArbitraryAxis=[0 0 1]  RotationSequenceAxes=FollowerAxes  RotationSequence=XYX  RotationSequenceAngles=[0 0 0]  RotationSequenceAnglesUnits=deg  RotationMatrix=[1 0 0; 0 1 0; 0 0 1]  Quaternion=[1 0 0 0]  TranslationMethod=None  TranslationCartesianOffset=[0 0 0]  TranslationCartesianOffsetUnits=m  TranslationStandardAxis=+Z  TranslationStandardOffset=0  TranslationStandardOffsetUnits=m  TranslationROffset=0  TranslationROffsetUnits=m  TranslationThetaOffset=0  TranslationThetaOffsetUnits=deg  TranslationZOffset=0  TranslationZOffsetUnits=m
  Transform Pos : sm_lib/Frames and Transforms/Rigid Transform  RotationMethod=StandardAxis  FollAlignAxisA=+X  BaseAlignAxisA=+Y  FollAlignAxisB=+Y  BaseAlignAxisB=+Z  RotationStandardAxis=-Y  RotationAngle=90  RotationAngleUnits=deg  RotationArbitraryAxis=[0 0 1]  RotationSequenceAxes=FollowerAxes  RotationSequence=XYX  RotationSequenceAngles=[0 0 0]  RotationSequenceAnglesUnits=deg  RotationMatrix=[1 0 0; 0 1 0; 0 0 1]  Quaternion=[1 0 0 0]  TranslationMethod=None  TranslationCartesianOffset=[0 0 0]  TranslationCartesianOffsetUnits=m  TranslationStandardAxis=+Z  TranslationStandardOffset=0  TranslationStandardOffsetUnits=m  TranslationROffset=0  TranslationROffsetUnits=m  TranslationThetaOffset=0  TranslationThetaOffsetUnits=deg  TranslationZOffset=0  TranslationZOffsetUnits=m
  Transform P1 : sm_lib/Frames and Transforms/Rigid Transform  RotationMethod=None  FollAlignAxisA=+X  BaseAlignAxisA=+Y  FollAlignAxisB=+Y  BaseAlignAxisB=+Z  RotationStandardAxis=+Z  RotationAngle=0.0  RotationAngleUnits=deg  RotationArbitraryAxis=[0 0 1]  RotationSequenceAxes=FollowerAxes  RotationSequence=XYX  RotationSequenceAngles=[0 0 0]  RotationSequenceAnglesUnits=deg  RotationMatrix=[1 0 0; 0 1 0; 0 0 1]  Quaternion=[1 0 0 0]  TranslationMethod=Cartesian  TranslationCartesianOffset=[(rad_drive+rad_ctr) -(rad_axis+rad_ctr) 0]  TranslationCartesianOffsetUnits=m  TranslationStandardAxis=+Y  TranslationStandardOffset=t_base_l/2  TranslationStandardOffsetUnits=m  TranslationROffset=0  TranslationROffsetUnits=m  TranslationThetaOffset=0  TranslationThetaOffsetUnits=deg  TranslationZOffset=0  TranslationZOffsetUnits=m
  Transform P3 : sm_lib/Frames and Transforms/Rigid Transform  RotationMethod=None  FollAlignAxisA=+X  BaseAlignAxisA=+Y  FollAlignAxisB=+Y  BaseAlignAxisB=+Z  RotationStandardAxis=+Z  RotationAngle=0.0  RotationAngleUnits=deg  RotationArbitraryAxis=[0 0 1]  RotationSequenceAxes=FollowerAxes  RotationSequence=XYX  RotationSequenceAngles=[0 0 0]  RotationSequenceAnglesUnits=deg  RotationMatrix=[1 0 0; 0 1 0; 0 0 1]  Quaternion=[1 0 0 0]  TranslationMethod=Cartesian  TranslationCartesianOffset=[-(rad_drive+rad_ctr) -(rad_axis+rad_ctr) 0]  TranslationCartesianOffsetUnits=m  TranslationStandardAxis=+Y  TranslationStandardOffset=t_base_l/2  TranslationStandardOffsetUnits=m  TranslationROffset=0  TranslationROffsetUnits=m  TranslationThetaOffset=0  TranslationThetaOffsetUnits=deg  TranslationZOffset=0  TranslationZOffsetUnits=m
  Transform P5 : sm_lib/Frames and Transforms/Rigid Transform  RotationMethod=None  FollAlignAxisA=+X  BaseAlignAxisA=+Y  FollAlignAxisB=+Y  BaseAlignAxisB=+Z  RotationStandardAxis=+Z  RotationAngle=0.0  RotationAngleUnits=deg  RotationArbitraryAxis=[0 0 1]  RotationSequenceAxes=FollowerAxes  RotationSequence=XYX  RotationSequenceAngles=[0 0 0]  RotationSequenceAnglesUnits=deg  RotationMatrix=[1 0 0; 0 1 0; 0 0 1]  Quaternion=[1 0 0 0]  TranslationMethod=Cartesian  TranslationCartesianOffset=[-(rad_drive+rad_ctr) (rad_axis+rad_ctr) 0]  TranslationCartesianOffsetUnits=m  TranslationStandardAxis=+Y  TranslationStandardOffset=t_base_l/2  TranslationStandardOffsetUnits=m  TranslationROffset=0  TranslationROffsetUnits=m  TranslationThetaOffset=0  TranslationThetaOffsetUnits=deg  TranslationZOffset=0  TranslationZOffsetUnits=m
  Transform P7 : sm_lib/Frames and Transforms/Rigid Transform  RotationMethod=None  FollAlignAxisA=+X  BaseAlignAxisA=+Y  FollAlignAxisB=+Y  BaseAlignAxisB=+Z  RotationStandardAxis=+Z  RotationAngle=0.0  RotationAngleUnits=deg  RotationArbitraryAxis=[0 0 1]  RotationSequenceAxes=FollowerAxes  RotationSequence=XYX  RotationSequenceAngles=[0 0 0]  RotationSequenceAnglesUnits=deg  RotationMatrix=[1 0 0; 0 1 0; 0 0 1]  Quaternion=[1 0 0 0]  TranslationMethod=Cartesian  TranslationCartesianOffset=[(rad_drive+rad_ctr) (rad_axis+rad_ctr) 0]  TranslationCartesianOffsetUnits=m  TranslationStandardAxis=+Y  TranslationStandardOffset=t_base_l/2  TranslationStandardOffsetUnits=m  TranslationROffset=0  TranslationROffsetUnits=m  TranslationThetaOffset=0  TranslationThetaOffsetUnits=deg  TranslationZOffset=0  TranslationZOffsetUnits=m
  P3 : PMIOPort  Side=Left
  P1 : PMIOPort  Port=2  Side=Left
  P5 : PMIOPort  Port=3  Side=Right
  B : PMIOPort  Port=4  Side=Left
  P7 : PMIOPort  Port=5  Side=Right
  P : PMIOPort  Port=6  Side=Right
  connections:
  P1/RConn1 -- Rod 1/RConn1
  Transform Base/LConn1 -- B/RConn1
  P5/RConn1 -- Rod 5/RConn1
  Slider/RConn1 -- Transform Base/RConn1
  P7/RConn1 -- Rod 7/RConn1
  Transform P1/LConn1 -- Transform P7/LConn1 -- Slider/LConn1 -- Transform P5/LConn1 -- Transform P3/LConn1 -- Transform Pos/LConn1
  P3/RConn1 -- Rod 3/RConn1
  P/RConn1 -- Transform Pos/RConn1
  Rod 3/LConn1 -- Transform P3/RConn1
  Rod 1/LConn1 -- Transform P1/RConn1
  Rod 5/LConn1 -- Transform P5/RConn1
  Rod 7/LConn1 -- Transform P7/RConn1

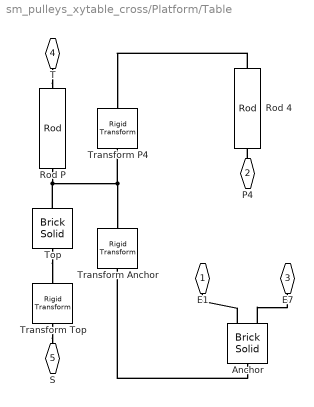
== system sm_pulleys_xytable_cross/Platform/Table ==
  Anchor : sm_lib/Body Elements/Brick Solid  BrickDimensions=[rad_axis/2 rad_axis*2 p_th]  BrickDimensionsUnits=m  ExportEntireGeometry=off  InertiaType=CalculateFromGeometry  BasedOnType=Density  Density=1000  DensityUnits=kg/m^3  Mass=1  MassUnits=kg  CenterOfMass=[0 0 0]  CenterOfMassUnits=m  MomentsOfInertia=[1 1 1]  MomentsOfInertiaUnits=kg*m^2  ProductsOfInertia=[0 0 0]  ProductsOfInertiaUnits=kg*m^2  GraphicType=FromGeometry  MarkerShape=Sphere  MarkerSize=10  GraphicVisPropType=SimpleVisualProperties  GraphicDiffuseColor=t_pos_clr  GraphicOpacity=1.0  GraphicSpecularColor=[0.5 0.5 0.5 1.0]  GraphicAmbientColor=[0.15 0.15 0.15 1.0]  GraphicEmissiveColor=[0.0 0.0 0.0 1.0]  GraphicShininess=75  DoExposeReferenceFrame=on  SerializedFrames=<Frames><Frame><Id>Frame1</Id><Value><Name>A</Name><Origin><Source>GeometricFeature</Source><FeatureName>-x -y curve</FeatureName></Origin><PrimaryAxis><DefinedDirection>+Z</DefinedDirection><Source>ReferenceFrame</Source><SourceDirection>+Z</SourceDirection><FeatureName></FeatureName></PrimaryAxis><SecondaryAxis><DefinedDirection>+X</DefinedDirection><Source>ReferenceFrame</Source><SourceDirection>+X</SourceDirection><FeatureName></FeatureName></SecondaryAxis></Value></Frame><Frame><Id>Frame2</Id><Value><Name>B</Name><Origin><Source>GeometricFeature</Source><FeatureName>-x +y curve</FeatureName></Origin><PrimaryAxis><DefinedDirection>+Z</DefinedDirection><Source>ReferenceFrame</Source><SourceDirection>+Z</SourceDirection><FeatureName></FeatureName></PrimaryAxis><SecondaryAxis><DefinedDirection>+X</DefinedDirection><Source>ReferenceFrame</Source><SourceDirection>+X</SourceDirection><FeatureName></FeatureName></SecondaryAxis></Value></Frame></Frames>
  Rod 4 : Multibody_Parts_Lib/Basic/Rod  rod_rad=p_hr  rod_len=p_th/2  rod_rho=7000  rod_color=[0.5 0.5 0.5]  rod_opc=1  popup_zori=Local +Z  popup_markings=None  mark_radius_range=[0.5 1.01]  mark_length_range=1.005  mark_angle_range=30  mark_color=[1 1 1]
      settings: SourceProductName=Simscape Multibody Parts Library
  Rod P : Multibody_Parts_Lib/Basic/Rod  rod_rad=p_hr  rod_len=p_th*2  rod_rho=7000  rod_color=[0.5 0.5 0.5]  rod_opc=1  popup_zori=Local +Z  popup_markings=None  mark_radius_range=[0.5 1.01]  mark_length_range=1.005  mark_angle_range=30  mark_color=[1 1 1]
      settings: SourceProductName=Simscape Multibody Parts Library
  Top : sm_lib/Body Elements/Brick Solid  BrickDimensions=[t_pos_w t_pos_l t_pos_h]  BrickDimensionsUnits=m  ExportEntireGeometry=off  InertiaType=CalculateFromGeometry  BasedOnType=Density  Density=1000  DensityUnits=kg/m^3  Mass=1  MassUnits=kg  CenterOfMass=[0 0 0]  CenterOfMassUnits=m  MomentsOfInertia=[1 1 1]  MomentsOfInertiaUnits=kg*m^2  ProductsOfInertia=[0 0 0]  ProductsOfInertiaUnits=kg*m^2  GraphicType=FromGeometry  MarkerShape=Sphere  MarkerSize=10  GraphicVisPropType=SimpleVisualProperties  GraphicDiffuseColor=t_pos_clr  GraphicOpacity=1.0  GraphicSpecularColor=[0.5 0.5 0.5 1.0]  GraphicAmbientColor=[0.15 0.15 0.15 1.0]  GraphicEmissiveColor=[0.0 0.0 0.0 1.0]  GraphicShininess=75  DoExposeReferenceFrame=off  SerializedFrames=<Frames><Frame><Id>Frame1</Id><Value><Name>T</Name><Origin><Source>GeometricFeature</Source><FeatureName>+z surface</FeatureName></Origin><PrimaryAxis><DefinedDirection>+Z</DefinedDirection><Source>ReferenceFrame</Source><SourceDirection>+Z</SourceDirection><FeatureName></FeatureName></PrimaryAxis><SecondaryAxis><DefinedDirection>+X</DefinedDirection><Source>ReferenceFrame</Source><SourceDirection>+X</SourceDirection><FeatureName></FeatureName></SecondaryAxis></Value></Frame><Frame><Id>Frame2</Id><Value><Name>B</Name><Origin><Source>GeometricFeature</Source><FeatureName>-z surface</FeatureName></Origin><PrimaryAxis><DefinedDirection>+Z</DefinedDirection><Source>ReferenceFrame</Source><SourceDirection>+Z</SourceDirection><FeatureName></FeatureName></PrimaryAxis><SecondaryAxis><DefinedDirection>+X</DefinedDirection><Source>ReferenceFrame</Source><SourceDirection>+X</SourceDirection><FeatureName></FeatureName></SecondaryAxis></Value></Frame></Frames>
  Transform Anchor : sm_lib/Frames and Transforms/Rigid Transform  RotationMethod=None  FollAlignAxisA=+X  BaseAlignAxisA=+Y  FollAlignAxisB=+Y  BaseAlignAxisB=+Z  RotationStandardAxis=+Z  RotationAngle=0.0  RotationAngleUnits=deg  RotationArbitraryAxis=[0 0 1]  RotationSequenceAxes=FollowerAxes  RotationSequence=XYX  RotationSequenceAngles=[0 0 0]  RotationSequenceAnglesUnits=deg  RotationMatrix=[1 0 0; 0 1 0; 0 0 1]  Quaternion=[1 0 0 0]  TranslationMethod=Cartesian  TranslationCartesianOffset=[(t_pos_w/2-rad_axis/4) 0 p_th/2]  TranslationCartesianOffsetUnits=m  TranslationStandardAxis=-X  TranslationStandardOffset=0  TranslationStandardOffsetUnits=m  TranslationROffset=0  TranslationROffsetUnits=m  TranslationThetaOffset=0  TranslationThetaOffsetUnits=deg  TranslationZOffset=0  TranslationZOffsetUnits=m
  Transform P4 : sm_lib/Frames and Transforms/Rigid Transform  RotationMethod=None  FollAlignAxisA=+X  BaseAlignAxisA=+Y  FollAlignAxisB=+Y  BaseAlignAxisB=+Z  RotationStandardAxis=+Z  RotationAngle=0.0  RotationAngleUnits=deg  RotationArbitraryAxis=[0 0 1]  RotationSequenceAxes=FollowerAxes  RotationSequence=XYX  RotationSequenceAngles=[0 0 0]  RotationSequenceAnglesUnits=deg  RotationMatrix=[1 0 0; 0 1 0; 0 0 1]  Quaternion=[1 0 0 0]  TranslationMethod=Cartesian  TranslationCartesianOffset=[-(t_pos_w/2-rad_axis) 0 0]  TranslationCartesianOffsetUnits=m  TranslationStandardAxis=-X  TranslationStandardOffset=0  TranslationStandardOffsetUnits=m  TranslationROffset=0  TranslationROffsetUnits=m  TranslationThetaOffset=0  TranslationThetaOffsetUnits=deg  TranslationZOffset=0  TranslationZOffsetUnits=m
  Transform Top : sm_lib/Frames and Transforms/Rigid Transform  RotationMethod=StandardAxis  FollAlignAxisA=+X  BaseAlignAxisA=+Y  FollAlignAxisB=+Y  BaseAlignAxisB=+Z  RotationStandardAxis=+Y  RotationAngle=90  RotationAngleUnits=deg  RotationArbitraryAxis=[0 0 1]  RotationSequenceAxes=FollowerAxes  RotationSequence=XYX  RotationSequenceAngles=[0 0 0]  RotationSequenceAnglesUnits=deg  RotationMatrix=[1 0 0; 0 1 0; 0 0 1]  Quaternion=[1 0 0 0]  TranslationMethod=None  TranslationCartesianOffset=[0 0 0]  TranslationCartesianOffsetUnits=m  TranslationStandardAxis=+Z  TranslationStandardOffset=0  TranslationStandardOffsetUnits=m  TranslationROffset=0  TranslationROffsetUnits=m  TranslationThetaOffset=0  TranslationThetaOffsetUnits=deg  TranslationZOffset=0  TranslationZOffsetUnits=m
  E1 : PMIOPort  Side=Left
  P4 : PMIOPort  Port=2  Side=Left
  E7 : PMIOPort  Port=3  Side=Left
  T : PMIOPort  Port=4  Side=Right
  S : PMIOPort  Port=5  Side=Right
  connections:
  P4/RConn1 -- Rod 4/RConn1
  Anchor/LConn1 -- E1/RConn1
  Anchor/RConn1 -- Transform Anchor/RConn1
  Anchor/LConn2 -- E7/RConn1
  Top/RConn1 -- Transform Top/RConn1
  Top/LConn1 -- Transform P4/LConn1 -- Transform Anchor/LConn1 -- Rod P/LConn1
  Transform Top/LConn1 -- S/RConn1
  Rod 4/LConn1 -- Transform P4/RConn1
  T/RConn1 -- Rod P/RConn1

== system sm_pulleys_xytable_cross/Pulleys/Peg2 ==
  Peg : sm_lib/Body Elements/Cylindrical Solid  CylinderRadius=p_hr  CylinderRadiusUnits=m  CylinderLength=p_th*4  CylinderLengthUnits=m  ExportEntireGeometry=off  InertiaType=CalculateFromGeometry  BasedOnType=Density  Density=1000  DensityUnits=kg/m^3  Mass=1  MassUnits=kg  CenterOfMass=[0 0 0]  CenterOfMassUnits=m  MomentsOfInertia=[1 1 1]  MomentsOfInertiaUnits=kg*m^2  ProductsOfInertia=[0 0 0]  ProductsOfInertiaUnits=kg*m^2  GraphicType=FromGeometry  MarkerShape=Sphere  MarkerSize=10  GraphicVisPropType=SimpleVisualProperties  GraphicDiffuseColor=[1 1 1]*0.95  GraphicOpacity=1.0  GraphicSpecularColor=[0.5 0.5 0.5 1.0]  GraphicAmbientColor=[0.15 0.15 0.15 1.0]  GraphicEmissiveColor=[0.0 0.0 0.0 1.0]  GraphicShininess=75  DoExposeReferenceFrame=off  SerializedFrames=<Frames><Frame><Id>Frame1</Id><Value><Name>B</Name><Origin><Source>GeometricFeature</Source><FeatureName>bottom surface</FeatureName></Origin><PrimaryAxis><DefinedDirection>+Z</DefinedDirection><Source>ReferenceFrame</Source><SourceDirection>+Z</SourceDirection><FeatureName></FeatureName></PrimaryAxis><SecondaryAxis><DefinedDirection>+X</DefinedDirection><Source>ReferenceFrame</Source><SourceDirection>+X</SourceDirection><FeatureName></FeatureName></SecondaryAxis></Value></Frame></Frames>
  Transform Peg : sm_lib/Frames and Transforms/Rigid Transform  RotationMethod=None  FollAlignAxisA=+X  BaseAlignAxisA=+Y  FollAlignAxisB=+Y  BaseAlignAxisB=+Z  RotationStandardAxis=+Z  RotationAngle=0.0  RotationAngleUnits=deg  RotationArbitraryAxis=[0 0 1]  RotationSequenceAxes=FollowerAxes  RotationSequence=XYX  RotationSequenceAngles=[0 0 0]  RotationSequenceAnglesUnits=deg  RotationMatrix=[1 0 0; 0 1 0; 0 0 1]  Quaternion=[1 0 0 0]  TranslationMethod=StandardAxis  TranslationCartesianOffset=[0 0 0]  TranslationCartesianOffsetUnits=m  TranslationStandardAxis=-X  TranslationStandardOffset=rad_drive*0.7  TranslationStandardOffsetUnits=m  TranslationROffset=0  TranslationROffsetUnits=m  TranslationThetaOffset=0  TranslationThetaOffsetUnits=deg  TranslationZOffset=0  TranslationZOffsetUnits=m
  B : PMIOPort  Side=Right
  connections:
  Transform Peg/LConn1 -- B/RConn1
  Peg/LConn1 -- Transform Peg/RConn1

== system sm_pulleys_xytable_cross/Pulleys/Peg6 ==
  Peg : sm_lib/Body Elements/Cylindrical Solid  CylinderRadius=p_hr  CylinderRadiusUnits=m  CylinderLength=p_th*4  CylinderLengthUnits=m  ExportEntireGeometry=off  InertiaType=CalculateFromGeometry  BasedOnType=Density  Density=1000  DensityUnits=kg/m^3  Mass=1  MassUnits=kg  CenterOfMass=[0 0 0]  CenterOfMassUnits=m  MomentsOfInertia=[1 1 1]  MomentsOfInertiaUnits=kg*m^2  ProductsOfInertia=[0 0 0]  ProductsOfInertiaUnits=kg*m^2  GraphicType=FromGeometry  MarkerShape=Sphere  MarkerSize=10  GraphicVisPropType=SimpleVisualProperties  GraphicDiffuseColor=[1 1 1]*0.95  GraphicOpacity=1.0  GraphicSpecularColor=[0.5 0.5 0.5 1.0]  GraphicAmbientColor=[0.15 0.15 0.15 1.0]  GraphicEmissiveColor=[0.0 0.0 0.0 1.0]  GraphicShininess=75  DoExposeReferenceFrame=off  SerializedFrames=<Frames><Frame><Id>Frame1</Id><Value><Name>B</Name><Origin><Source>GeometricFeature</Source><FeatureName>bottom surface</FeatureName></Origin><PrimaryAxis><DefinedDirection>+Z</DefinedDirection><Source>ReferenceFrame</Source><SourceDirection>+Z</SourceDirection><FeatureName></FeatureName></PrimaryAxis><SecondaryAxis><DefinedDirection>+X</DefinedDirection><Source>ReferenceFrame</Source><SourceDirection>+X</SourceDirection><FeatureName></FeatureName></SecondaryAxis></Value></Frame></Frames>
  Transform Peg : sm_lib/Frames and Transforms/Rigid Transform  RotationMethod=None  FollAlignAxisA=+X  BaseAlignAxisA=+Y  FollAlignAxisB=+Y  BaseAlignAxisB=+Z  RotationStandardAxis=+Z  RotationAngle=0.0  RotationAngleUnits=deg  RotationArbitraryAxis=[0 0 1]  RotationSequenceAxes=FollowerAxes  RotationSequence=XYX  RotationSequenceAngles=[0 0 0]  RotationSequenceAnglesUnits=deg  RotationMatrix=[1 0 0; 0 1 0; 0 0 1]  Quaternion=[1 0 0 0]  TranslationMethod=StandardAxis  TranslationCartesianOffset=[0 0 0]  TranslationCartesianOffsetUnits=m  TranslationStandardAxis=-X  TranslationStandardOffset=rad_drive*0.7  TranslationStandardOffsetUnits=m  TranslationROffset=0  TranslationROffsetUnits=m  TranslationThetaOffset=0  TranslationThetaOffsetUnits=deg  TranslationZOffset=0  TranslationZOffsetUnits=m
  B : PMIOPort  Side=Right
  connections:
  Peg/LConn1 -- Transform Peg/RConn1
  Transform Peg/LConn1 -- B/RConn1

== system sm_pulleys_xytable_cross/Pulleys/Revolute P2 ==
  Actuate : Subsystem  VariantControl=Actuate
      mask Display: image('sm_pulleys_xytable_cross_pulleyAnglesActuate_IMAGE.png');
  Measure : Subsystem  VariantControl=Measure
      mask Display: image('sm_pulleys_xytable_cross_pulleyAnglesMeasure_IMAGE.png');
  " B" : PMIOPort  Side=Left
  " F" : PMIOPort  Port=2  Side=Right

== system sm_pulleys_xytable_cross/Pulleys/Revolute P6 ==
  Actuate : Subsystem  Tag=PublishSubsystem  VariantControl=Actuate
      mask Display: image('sm_pulleys_xytable_cross_pulleyAnglesActuate_IMAGE.png');
  Measure : Subsystem  Tag=PublishSubsystem  VariantControl=Measure
      mask Display: image('sm_pulleys_xytable_cross_pulleyAnglesMeasure_IMAGE.png');
  " F" : PMIOPort  Side=Right
  " B" : PMIOPort  Port=2  Side=Left
